simulink model "e8_PMSM_SprayMultiNozzle_ROM"  (R2021b)
settings: Solver=VariableStepAuto  StartTime=0.0  StopTime=1000  RelTol=1e-3  AbsTol=1e-3
model workspace (MAT data in the model file):
  AdjacencyMat = [0 0 0 0 0 0 0 0 0 0 0 0 ... (12996 elements, 114x114)]
  Banding_Loss_Mat = [0 0 0 0 0 0 0 0 0 0 0 0 ... (2340 elements, 39x60)]
  CapMat = [1e+20; 2196.70091586; 387.653102799; 193.8265514; 1962.34710525; 387.653102799; 193.8265514; 1962.34710525; 1266.59353814; 268.053957132; 416.539515956; 175.715078; 577.243160678; 310.101557898; 23.9530731873; 15.4990473565; 47.9061463746; 30.998094713; 1.17508343445; 1.17508343445; 86.96376; 450.202206395; 54.9511679003; 54.9511679003; 247.389926005; 247.389926005; 75.306462; 75.306462; 1e+20; 1e+20; 1e+20; 1e+20; 1e+20; 0; 0; 0; 0; 429.469897824; 0; 0; 0; 0; 429.469897824; 0; 0; 0; 0; 0; 0; 424.408023296; 268.053957132; 0; 0; 0; 0; 0; 322.102423368; 0; 0; 0; 0; 0; 322.102423368; 0; 0; 0; 0; 0; 318.306017472; 268.053957132; 2196.70091586; 1266.59353814; 268.053957132; 416.539515956; 175.715078; 577.243160678; 310.101557898; 86.96376; 450.202206395; 0; 0; 0; 0; 0; 424.408023296; 268.053957132; 0; 0; 0; 0; 318.306017472; 268.053957132; 2196.70091586; 1266.59353814; 268.053957132; 416.539515956; 175.715078; 577.243160678; 310.101557898; 86.96376; 450.202206395; 0; 0; 0; 0; 0; 424.408023296; 268.053957132; 0; 0; 0; 0; 318.306017472; 268.053957132]
  CoolantArrayIdxs = [21; 29; 78; 100; 30; 31; 32; 33]
  Friction_Loss_Mat = [0 0 0 0 0 0 0 0 0 0 0 0 ... (2340 elements, 39x60)]
  InletCoolIdxs = [30  31  32  33; 29  29  29  29; 30  31  32  33]
  Iron_Loss_Rotor_Back_Iron_Mat = [0.0117705351991 0.0200087653806 0.0246811430764 0.0256578010281 0.0240025552689 0.0207013457731 0.0167627779958 0.013305715839 0.0115602539828 0.0121149481083 0.0143511671725 0.0171856755847 ... (2340 elements, 39x60)]
  Iron_Loss_Rotor_Pole_Mat = [1.45649756865 1.45241481649 1.42884898554 1.39022048903 1.34148134724 1.28634015611 1.22776297278 1.16827194649 1.11002512364 1.05393003616 0.999091137463 0.943664155592 ... (2340 elements, 39x60)]
  Iron_Loss_Rotor_Tooth_Mat = [0 0 0 0 0 0 0 0 0 0 0 0 ... (2340 elements, 39x60)]
  Iron_Loss_Stator_Back_Iron_Mat = [38.5419456951 37.7562377622 36.7626331345 35.6659256425 34.5041164064 33.3097183676 32.1148301022 30.9550268851 29.8690226279 28.862614511 27.8706329494 26.7877765024 ... (2340 elements, 39x60)]
  Iron_Loss_Stator_Tooth_Mat = [42.0610884508 41.0367236596 40.1636589805 39.4141834911 38.6901612332 37.9457147976 37.1698474109 36.3762859147 35.5917582202 34.8149830437 33.9858111542 33.0265171037 ... (2340 elements, 39x60)]
  LossDistrForEachType = [0 0 0 0 0 0 0 0 0 0 0 0 ... (2736 elements, 24x114)]
  Magnet_Loss_Mat = [0.0995193918038 0.0927324879203 0.0867464499603 0.0817901209144 0.0773904805464 0.0731587227427 0.068708638331 0.0635818407139 0.057217354686 0.0494585613633 0.0409403305493 0.0325683424692 ... (2340 elements, 39x60)]
  OutletCoolIdxs = [30  31  32  33; 100  100  100  100; 30  31  32  33]
  RotorCopperTempCoefResistivity = 0.00393
  Rotor_Cage_Loss_Mat = [0 0 0 0 0 0 0 0 0 0 0 0 ... (2340 elements, 39x60)]
  ShaftTorqueVec = [-286.936099977 -271.951133863 -256.966167748 -241.981201634 -226.99623552 -212.011269406 -197.026303292 -182.041337178 -167.056371063 -152.071404949 -137.086438835 -122.101472721 -107.116506607 -92.1315404924 -77.1465743783 -62.1616082641 -47.1766421499 -32.1916760357 -17.2067099215 -2.22174380736 12.7632223068 27.748188421 42.7331545352 57.7181206494 72.7030867635 87.6880528777 102.673018992 117.657985106 132.64295122 147.627917334 162.612883449 177.597849563 192.582815677 207.567781791 222.552747905 237.53771402 252.522680134 267.507646248 282.492612362]
  Sleeve_Loss_Mat = [0 0 0 0 0 0 0 0 0 0 0 0 ... (2340 elements, 39x60)]
  SpeedVec = [500 661.016949153 822.033898305 983.050847458 1144.06779661 1305.08474576 1466.10169492 1627.11864407 1788.13559322 1949.15254237 2110.16949153 2271.18644068 2432.20338983 2593.22033898 2754.23728814 2915.25423729 3076.27118644 3237.28813559 3398.30508475 3559.3220339 3720.33898305 3881.3559322 4042.37288136 4203.38983051 4364.40677966 4525.42372881 4686.44067797 4847.45762712 5008.47457627 5169.49152542 5330.50847458 5491.52542373 5652.54237288 5813.55932203 5974.57627119 6135.59322034 6296.61016949 6457.62711864 6618.6440678 6779.66101695 6940.6779661 7101.69491525 7262.71186441 7423.72881356 7584.74576271 7745.76271186 7906.77966102 8067.79661017 8228.81355932 8389.83050847 8550.84745763 8711.86440678 8872.88135593 9033.89830508 9194.91525424 9355.93220339 9516.94915254 9677.96610169 9838.98305085 10000]
  StateSpaceND : object (value not decoded)
  StatorCopperTempCoefResistivity = 0.00393
  Stator_Copper_Loss_AC_Mat = [0 0 0 0 0 0 0 0 0 0 0 0 ... (2340 elements, 39x60)]
  Stator_Copper_Loss_Mat = [3925.33912093 3500.33132705 3080.91358293 2704.55804144 2364.73307434 2056.62848353 1776.61435032 1521.89015388 1290.25886694 1079.99319182 889.737399072 718.403752767 ... (2340 elements, 39x60)]
  Stray_Load_Loss_Mat = [0 0 0 0 0 0 0 0 0 0 0 0 ... (2340 elements, 39x60)]
  Stray_Loss_Stator_Iron_Proportion = 0.95
  TnodesInit = [25; 25; 25; 25; 25; 25; 25; 25; 25; 25; 25; 25; 25; 25; 25; 25; 25; 25; 25; 25; 25; 25; 25; 25; 25; 25; 25; 25; 25; 25; 25; 25; 25; 25; 25; 25; 25; 25; 25; 25; 25; 25; 25; 25; 25; 25; 25; 25; 25; 25; 25; 25; 25; 25; 25; 25; 25; 25; 25; 25; 25; 25; 25; 25; 25; 25; 25; 25; 25; 25; 25; 25; 25; 25; 25; 25; 25; 25; 25; 25; 25; 25; 25; 25; 25; 25; 25; 25; 25; 25; 25; 25; 25; 25; 25; 25; 25; 25; 25; 25; 25; 25; 25; 25; 25; 25; 25; 25; 25; 25; 25; 25; 25; 25]
  TrefRotor = 20
  TrefStator = 20
  Windage_Loss_Mat = [0 0 0 0 0 0 0 0 0 0 0 0 ... (2340 elements, 39x60)]
libraries: mcadROM_lib x4
(part 1 of 2)
settings Model: Creator=agonzale  LastModifiedBy=agonzale
settings SolverCC: AutoScaleAbsTol=off

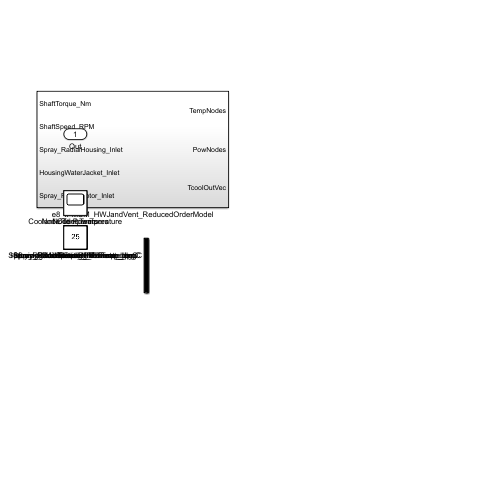
[thumbnail: Simulink's stored preview of the top-level diagram]
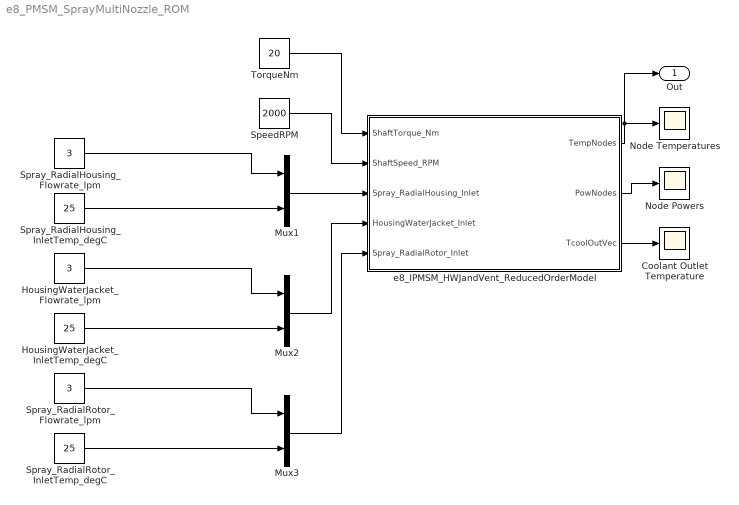
== system e8_PMSM_SprayMultiNozzle_ROM ==
  Coolant Outlet Temperature : Scope
  HousingWaterJacket_Flowrate_lpm : Constant  Value=3
  HousingWaterJacket_InletTemp_degC : Constant  Value=25
  Mux1 : Mux  Inputs=2
  Mux2 : Mux  Inputs=2
  Mux3 : Mux  Inputs=2
  Node Powers : Scope
  Node Temperatures : Scope
  SpeedRPM : Constant  Value=2000
  Spray_RadialHousing_Flowrate_lpm : Constant  Value=3
  Spray_RadialHousing_InletTemp_degC : Constant  Value=25
  Spray_RadialRotor_Flowrate_lpm : Constant  Value=3
  Spray_RadialRotor_InletTemp_degC : Constant  Value=25
  TorqueNm : Constant  Value=20
  e8_IPMSM_HWJandVent_ReducedOrderModel : Subsystem
  Out : Outport
  wires:
  HousingWaterJacket_InletTemp_degC/1 -> Mux2/2
  HousingWaterJacket_Flowrate_lpm/1 -> Mux2/1
  e8_IPMSM_HWJandVent_ReducedOrderModel/3(TcoolOutVec) -> Coolant Outlet Temperature/1
  e8_IPMSM_HWJandVent_ReducedOrderModel/2(PowNodes) -> Node Powers/1
  Mux3/1 -> e8_IPMSM_HWJandVent_ReducedOrderModel/5(Spray_RadialRotor_Inlet)
  Spray_RadialRotor_InletTemp_degC/1 -> Mux3/2
  Spray_RadialRotor_Flowrate_lpm/1 -> Mux3/1
  Mux2/1 -> e8_IPMSM_HWJandVent_ReducedOrderModel/4(HousingWaterJacket_Inlet)
  Mux1/1 -> e8_IPMSM_HWJandVent_ReducedOrderModel/3(Spray_RadialHousing_Inlet)
  Spray_RadialHousing_Flowrate_lpm/1 -> Mux1/1
  Spray_RadialHousing_InletTemp_degC/1 -> Mux1/2
  SpeedRPM/1 -> e8_IPMSM_HWJandVent_ReducedOrderModel/2(ShaftSpeed_RPM)
  TorqueNm/1 -> e8_IPMSM_HWJandVent_ReducedOrderModel/1(ShaftTorque_Nm)
  e8_IPMSM_HWJandVent_ReducedOrderModel/1(TempNodes) -> Node Temperatures/1, Out/1
